simulink model "rest_spike_bistability"  (R2015a)
settings: Solver=ode45  StartTime=0.0  StopTime=10000  RelTol=1e-3
values from neighbouring files (symbols this model uses):
  alpha = a(i)    [AsymOscillPeriods.m]    (also in averagedRelayOutput.m = alphaArray(i); bursting_linearised.m = 0.5; compareApproximations.m = 0.5; evaluateDerivatives.m = variables(3))
  beta = 0.37    [averagedRelayOutput.m]    (also in bursting_linearised.m = 0.27; compareApproximations.m = 1.5; fastSlow.m; fast_nullcline_winged_cusp.m = 0.5)
  delta = 0.5    [averagedRelayOutput.m]    (also in bursting_linearised.m; compareApproximations.m; fastSlow.m; fast_nullcline_winged_cusp.m)
  gamma = 0    [averagedRelayOutput.m]    (also in bursting_linearised.m = 1; compareApproximations.m = 1; fastSlow.m; fast_nullcline_winged_cusp.m = 1)
  ts = 1    [averagedRelayOutput.m]    (also in bursting_linearised.m; compareApproximations.m; fastSlow.m; fast_nullcline_winged_cusp.m)
settings Model: CovModelRefEnable=off  Creator=rajiv  LastModifiedBy=rajiv
settings DataIOCC: SaveFormat=Dataset
settings HardwareCC: ProdBitPerPointer=64  ProdLargestAtomicFloat=Float  ProdIntDivRoundTo=Zero  ProdEndianess=LittleEndian  ProdHWDeviceType=Specified
settings GRTTargetCC: GeneratePreprocessorConditionals=Use local settings

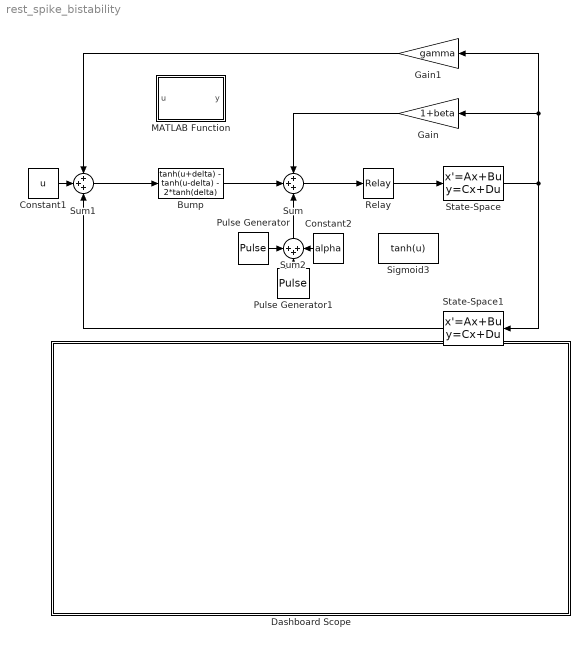
== system rest_spike_bistability ==
  Bump : Fcn  Expr="tanh(u+delta) -  tanh(u-delta) - 2*tanh(delta)"
  Constant1 : Constant  Value=u
  Constant2 : Constant  Value=alpha
  Dashboard Scope : Subsystem  DialogController=hmiCreateDDGDialog  IsWebBlock=on  mask(MWDashboardBlock){webBlockId=68aa9a0c-b9c9-4419-83a5-8653b2e17286, webBlockType=sdiscope, ShowInitialText=on, HMISrcModelName=rest_spike_bistability}
      mask prompts: webBlockId "WebBlock Id"; webBlockType "WebBlock Type"; HMISrcModelName "Source Model"
      mask Help: helpview([docroot '/mapfiles/simulink.map'], 'hmi_scope')
      mask Display:
      | if strcmp(get_param(bdroot(gcb),'BlockDiagramType'), 'library')
      |     image([(matlabroot) '/toolbox/simulink/hmi/icons/DashboardScope.png']);
      | end
  Gain : Gain  Gain=1+beta
  Gain1 : Gain  Gain=gamma
  MATLAB Function : MATLAB Function  TreatAsAtomicUnit=on
      settings: PermitHierarchicalResolution=ParametersOnly
  Pulse Generator : DiscretePulseGenerator  PulseType=Time based  Amplitude=2  Period=10000  PhaseDelay=4000
  Pulse Generator1 : DiscretePulseGenerator  PulseType=Time based  Amplitude=-2  Period=10000  PhaseDelay=7000
  Relay : Relay  OnSwitchValue=0  OffSwitchValue=0  OffOutputValue=-1
  Sigmoid3 : Fcn  Expr=tanh(u)
  State-Space : StateSpace  A=-1/tf  B=1/tf  D=0  X0=-1
  State-Space1 : StateSpace  A=-1/ts  B=1/ts  D=0  X0=-1
  Sum : Sum  Inputs=+++
  Sum1 : Sum  Inputs=+++
  Sum2 : Sum  Inputs=+++
  wires:
  Sum/1 -> Relay/1
  Gain/1 -> Sum/1
  State-Space1/1 -> Sum1/3
  Gain1/1 -> Sum1/1
  Constant1/1 -> Sum1/2
  Relay/1 -> State-Space/1
  State-Space/1 -> State-Space1/1, Gain/1, Gain1/1
  Constant2/1 -> Sum2/3
  Pulse Generator/1 -> Sum2/1
  Sum2/1 -> Sum/3
  Pulse Generator1/1 -> Sum2/2
  Bump/1 -> Sum/2
  Sum1/1 -> Bump/1

== system rest_spike_bistability/Dashboard Scope ==

== matlab function rest_spike_bistability/MATLAB Function ==
  data: u input; y output
function y = fcn(u)
%#codegen
if (u < -2)
    y = -1;
elseif (u > 2)
    y = -1;
elseif and( u>=-2,u < 0)
    y = 0.5*u;
else
    y = -0.5*u;
end
